simulink model "resistenciaBacteriasPulseTrain"  (R2017a)
settings: Solver=VariableStepAuto  StartTime=0.0  StopTime=1000.0  MaxStep=0.05  RelTol=1e-3
libraries: simulink x3
settings Model: Creator=posoriol1  LastModifiedBy=pablo

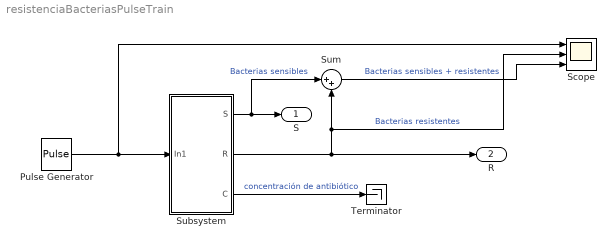
== system resistenciaBacteriasPulseTrain ==
  Pulse Generator : DiscretePulseGenerator  PulseType=Time based  Amplitude=.5  Period=50  PulseWidth=5
  Scope : Scope  NumInputPorts=3
  Subsystem : Subsystem  mask{par=[0.14 0.1 0.3960 4^(-3) 0.2 0.09 0.0083], x0=[0.2 0 1]}
      mask prompts: par "[bs br alphas q ms mr mc]"; x0 "Cond iniciales (s0,r0,c0)"
      mask init:
      | bs=par(1);br=par(2);alphas=par(3);q=par(4);ms=par(5);mr=par(6);mc=par(7);
  Sum : Sum  Inputs=|++
  Terminator : Terminator
  S : Outport
  R : Outport  Port=2
  wires:
  Subsystem/1(S) -> Sum/1, S/1  "Bacterias sensibles"
  Sum/1 -> Scope/3  "Bacterias sensibles + resistentes"
  Subsystem/2(R) -> R/1, Scope/2, Sum/2  "Bacterias resistentes"
  Subsystem/3("C ") -> Terminator/1  "concentración de antibiótico"
  Pulse Generator/1 -> Scope/1, Subsystem/1(In1)

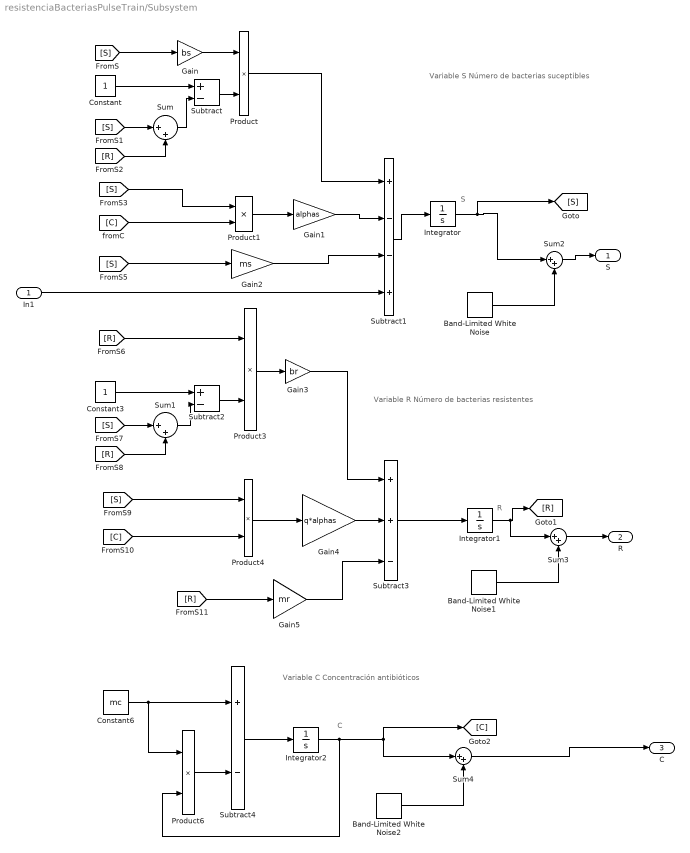
== system resistenciaBacteriasPulseTrain/Subsystem ==
  note: C
  note: Variable C
      | Concentración antibióticos
  note: R
  note: S
  note: Variable S
      | Número de bacterias suceptibles
  note: Variable R
      | Número de bacterias resistentes
  In1 : Inport
  Band-Limited White Noise : simulink/Sources/Band-Limited White Noise  Cov=[0.0000001]  Ts=0.1  seed=[23341]
  Band-Limited White Noise1 : simulink/Sources/Band-Limited White Noise  Cov=[0.0000005]  Ts=0.1  seed=[12341]
  Band-Limited White Noise2 : simulink/Sources/Band-Limited White Noise  Cov=[0.0000005]  Ts=0.1  seed=[13458]
  Constant : Constant
  Constant3 : Constant
  Constant6 : Constant  Value=mc
  Gain : Gain  Gain=bs
  Gain1 : Gain  Gain=alphas
  Gain2 : Gain  Gain=ms
  Gain3 : Gain  Gain=br
  Gain4 : Gain  Gain=q*alphas
  Gain5 : Gain  Gain=mr
  Integrator : Integrator  InitialCondition=x0(1)
  Integrator1 : Integrator  InitialCondition=x0(2)
  Integrator2 : Integrator  InitialCondition=x0(3)
  Product{,1,3..4,6} (5 alike) : Product
  Subtract : Sum  Inputs=+-
  Subtract1 : Sum  Inputs=+--+
  Subtract2 : Sum  Inputs=+-
  Subtract3 : Sum  Inputs=++-
  Subtract4 : Sum  Inputs=+-
  Sum{,1..4} (5 alike) : Sum  Inputs=|++
  S : Outport
  R : Outport  Port=2
  "C " : Outport  Port=3
  wires:
  [S] -> Sum/1
  [R] -> Sum/2
  Constant/1 -> Subtract/1
  [S] -> Sum1/1
  Sum1/1 -> Subtract2/2
  Subtract1/1 -> Integrator/1
  Integrator/1 -> [S], Sum2/1
  [R] -> Sum1/2
  Product4/1 -> Gain4/1
  Constant3/1 -> Subtract2/1
  Product3/1 -> Gain3/1
  Product/1 -> Subtract1/1
  Integrator1/1 -> Sum3/1, [R]
  Subtract3/1 -> Integrator1/1
  Sum/1 -> Subtract/2
  Integrator2/1 -> Product6/2, Sum4/1, [C]
  Subtract4/1 -> Integrator2/1
  Product6/1 -> Subtract4/2
  Constant6/1 -> Product6/1, Subtract4/1
  [S] -> Gain/1
  Gain/1 -> Product/1
  Subtract/1 -> Product/2
  Product1/1 -> Gain1/1
  Gain1/1 -> Subtract1/2
  [S] -> Product1/1
  [C] -> Product1/2
  [S] -> Gain2/1
  Gain2/1 -> Subtract1/3
  Gain3/1 -> Subtract3/1
  [R] -> Product3/1
  Subtract2/1 -> Product3/2
  Gain4/1 -> Subtract3/2
  [S] -> Product4/1
  [C] -> Product4/2
  Gain5/1 -> Subtract3/3
  [R] -> Gain5/1
  In1/1 -> Subtract1/4
  Sum2/1 -> S/1
  Band-Limited White Noise/1 -> Sum2/2
  Band-Limited White Noise1/1 -> Sum3/2
  Sum3/1 -> R/1
  Band-Limited White Noise2/1 -> Sum4/2
  Sum4/1 -> "C "/1
